simulink model "pos2airgapUNITS"  (R2022b)
settings: Solver=FixedStepAuto  StartTime=0.0  StopTime=10.0  RelTol=1e-3
settings Model: Creator=USUARIO  LastModifiedBy=ramuj

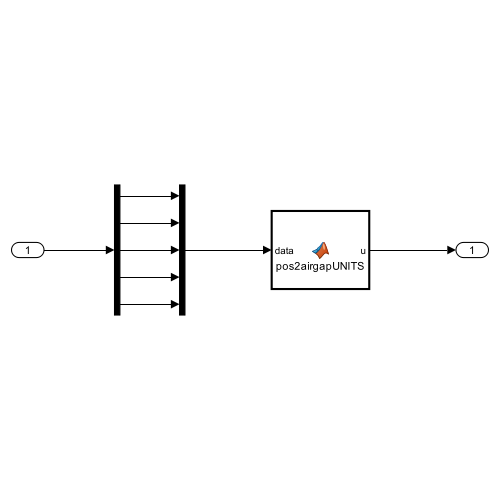
[thumbnail: Simulink's stored preview of the top-level diagram]
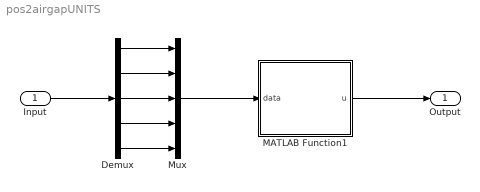
== system pos2airgapUNITS ==
  Input : Inport  SampleTime=1/7500
  Demux : Demux  Outputs=5
  MATLAB Function1 : MATLAB Function  TreatAsAtomicUnit=on
  Mux : Mux  Inputs=5
  Output : Outport
  wires:
  Demux/1 -> Mux/1
  Demux/2 -> Mux/2
  Demux/5 -> Mux/5
  Demux/3 -> Mux/3
  Mux/1 -> MATLAB Function1/1(data)
  Demux/4 -> Mux/4
  Input/1 -> Demux/1
  MATLAB Function1/1(u) -> Output/1

== matlab function pos2airgapUNITS/MATLAB Function1 ==
  data: data input; u output
function u = pos2airgapUNITS(data)

% CONSTANTES
x_ems = 0.49667;
y_ems = 0.268;
z_ems = -0.04113;
x_hems = 0.4925;
y_hems = 0.23675;
z_hems = 0.05299;
z_infr = 0.6328;
y_infr = 0.280;

y = data(1);
z = data(2);
rotx = data(3);
roty = data(4);
rotz = data(5);

grosory = 0.005;
grosorz = 0.015;

% DISTANCIAS
airgap5 = y_infr - y_ems * cos(rotz) - y - x_ems * sin(rotz) + z_ems * sin(rotx);
airgap6 = y_infr - y_ems * cos(rotz) + y + x_ems * sin(rotz) - z_ems * sin(rotx);
airgap7 = y_infr - y_ems * cos(rotz) - y + x_ems * sin(rotz) + z_ems * sin(rotx);
airgap8 = y_infr - y_ems * cos(rotz) + y - x_ems * sin(rotz) - z_ems * sin(rotx);

airgap1 =  +z - z_infr  + z_hems * cos(roty) - x_hems * sin(roty) + y_hems * sin(rotx) - grosorz;
airgap2 =  +z - z_infr  + z_hems * cos(roty) - x_hems * sin(roty) - y_hems * sin(rotx) - grosorz;
airgap3 =  +z - z_infr  + z_hems * cos(roty) + x_hems * sin(roty) + y_hems * sin(rotx) - grosorz;
airgap4 =  +z - z_infr  + z_hems * cos(roty) + x_hems * sin(roty) - y_hems * sin(rotx) - grosorz;

u =[airgap1, airgap2, airgap3, airgap4, airgap5, airgap6, airgap7, airgap8]';
